simulink model "Mass_Damper_Sys"  (R2024a)
settings: Solver=VariableStepAuto  StartTime=0.0  StopTime=10.0  RelTol=1e-3
settings Model: Creator=VICTUS  LastModifiedBy=VICTUS

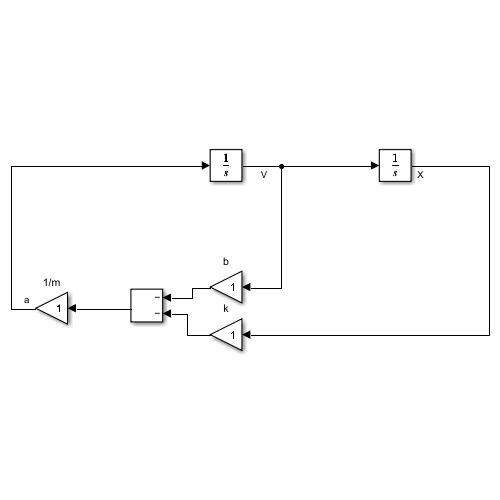
[thumbnail: Simulink's stored preview of the top-level diagram]
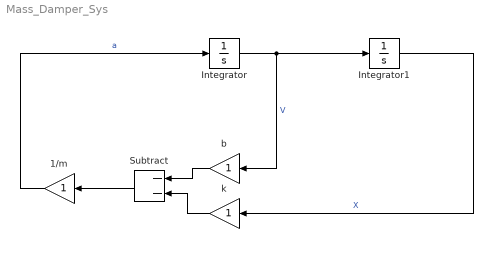
== system Mass_Damper_Sys ==
  1/m : Gain
  Integrator : Integrator
  Integrator1 : Integrator
  Subtract : Sum  Inputs=--
  b : Gain
  k : Gain
  wires:
  Integrator/1 -> b/1, Integrator1/1  "V"
  Integrator1/1 -> k/1  "X"
  b/1 -> Subtract/1
  k/1 -> Subtract/2
  Subtract/1 -> 1/m/1
  1/m/1 -> Integrator/1  "a"
